simulink model "Farrow2"  (R2022b)
settings: Solver=VariableStepAuto  StartTime=0.0  StopTime=10.0  RelTol=1e-3
values from neighbouring files (symbols this model uses):
  C = [-0.1667, 0.5, -0.3333, 0 ... (first row only)    [Fractional Delay Filter.m]
  Delta = 0.5    [Fractional Delay Filter.m]
  Ts = 1/fs    (= 0.001)    [Fractional Delay Filter.m]
settings Model: Creator=josef  LastModifiedBy=m.haris
settings DataIOCC: ReturnWorkspaceOutputs=off
settings DebuggingCC: UnconnectedInputMsg=warning  UnconnectedOutputMsg=warning  UnconnectedLineMsg=warning
settings ModelReferenceCC: EnableRefExpFcnMdlSchedulingChecks=on
settings RTWCC: DLArmComputeVersion=19.05

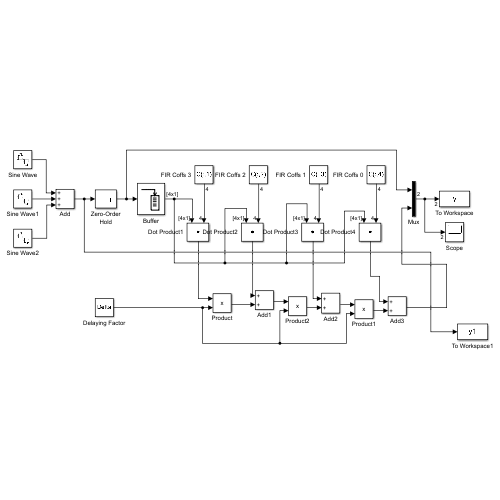
[thumbnail: Simulink's stored preview of the top-level diagram]
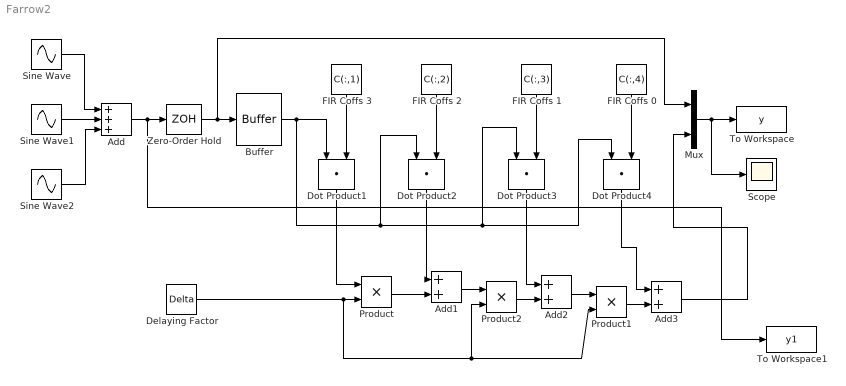
== system Farrow2 ==
  Add : Sum  Inputs=+++
  Add1 : Sum
  Add2 : Sum
  Add3 : Sum
  Buffer : Buffer  N=4  V=3  OutputFrames=off
  Delaying Factor : Constant  Value=Delta
  Dot Product{1..4} (4 alike) : DotProduct  OutDataTypeStr=Inherit: Inherit via internal rule
  FIR Coffs 0 : Constant  Value=C(:,4)
  FIR Coffs 1 : Constant  Value=C(:,3)
  FIR Coffs 2 : Constant  Value=C(:,2)
  FIR Coffs 3 : Constant  Value=C(:,1)
  Mux : Mux  Inputs=2
  Product : Product
  Product1 : Product
  Product2 : Product
  Scope : Scope
  Sine Wave : Sin  Frequency=2*pi*10  SampleTime=Ts/100
  Sine Wave1 : Sin  Frequency=2*pi*50  SampleTime=Ts/100
  Sine Wave2 : Sin  Frequency=2*pi*100  SampleTime=Ts/100
  To Workspace : ToWorkspace  VariableName=y  SaveFormat=Timeseries  SampleTime=-1
  To Workspace1 : ToWorkspace  VariableName=y1  SaveFormat=Timeseries  SampleTime=-1
  Zero-Order Hold : ZeroOrderHold  SampleTime=Ts
  wires:
  Sine Wave2/1 -> Add/3
  Sine Wave1/1 -> Add/2
  Sine Wave/1 -> Add/1
  Add/1 -> To Workspace1/1, Zero-Order Hold/1
  Zero-Order Hold/1 -> Buffer/1, Mux/1
  Mux/1 -> To Workspace/1, Scope/1
  FIR Coffs 3/1 -> Dot Product1/2
  FIR Coffs 2/1 -> Dot Product2/2
  Buffer/1 -> Dot Product4/1, Dot Product3/1, Dot Product2/1, Dot Product1/1
  FIR Coffs 1/1 -> Dot Product3/2
  FIR Coffs 0/1 -> Dot Product4/2
  Add3/1 -> Mux/2
  Dot Product3/1 -> Add2/1
  Dot Product1/1 -> Product/1
  Product2/1 -> Add2/2
  Dot Product2/1 -> Add1/1
  Add2/1 -> Product1/1
  Add1/1 -> Product2/1
  Product1/1 -> Add3/2
  Delaying Factor/1 -> Product1/2, Product2/2, Product/2
  Dot Product4/1 -> Add3/1
  Product/1 -> Add1/2
